simulink model "thirdweek_first"  (R2020a)
settings: Solver=VariableStepAuto  StartTime=0.0  StopTime=10.0  RelTol=1e-3
settings Model: Creator=Admin  LastModifiedBy=Admin

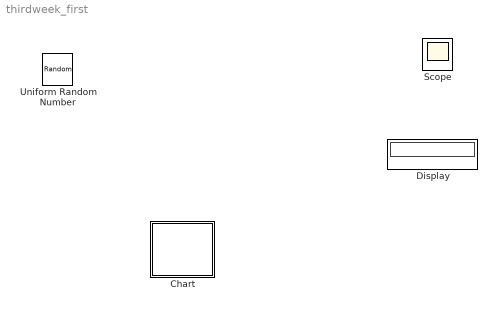
== system thirdweek_first ==
  Chart : Stateflow chart  TreatAsAtomicUnit=on
  Display : Display
  Scope : Scope
  Uniform Random Number : UniformRandomNumber  Minimum=0  Maximum=2  Seed=250  SampleTime=10

== stateflow chart thirdweek_first/Chart ==
  state No_Money
  (default) -> No_Money
